simulink model "simulink_audiotest"  (Simulink 7.6)
settings: Solver=ode3  StartTime=0.0  StopTime=100.0  RelTol=1e-3
libraries: dspsrcs4 x3, dspsnks4 x2, simulink x1
settings Model: Creator=KBE  LastModifiedBy=kbe
settings OptimizationCC: InitFltsAndDblsToZero=on
settings DebuggingCC: StrictBusMsg=Warning

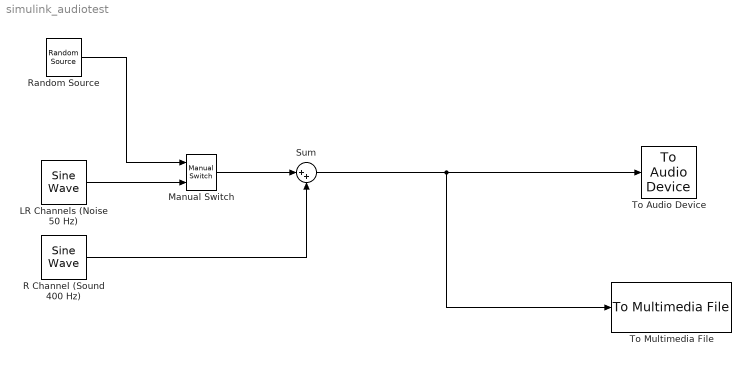
== system simulink_audiotest ==
  LR Channels (Noise 50 Hz) : dspsrcs4/Sine Wave  Amplitude=[1 1]  Frequency=[100 100]  Phase=[0 0]  SampleMode=Discrete  OutComplex=Real  CompMethod=Trigonometric fcn  TableSize=Speed  SampleTime=1/1000  SamplesPerFrame=1  ResetState=Restart at time zero  dataType=double  wordLen=16  udDataType=sfix(16)  fracBitsMode=Best precision  numFracBits=15  OutDataTypeStr=double  LastOutDataTypeStr=double
  Manual Switch : simulink/Signal Routing/Manual Switch  SystemSampleTime=-1  sw=0  action=0  varsize=off
  R Channel (Sound 400 Hz) : dspsrcs4/Sine Wave  Amplitude=[0 1]  Frequency=[400 400]  Phase=[0 0]  SampleMode=Discrete  OutComplex=Real  CompMethod=Trigonometric fcn  TableSize=Speed  SampleTime=1/1000  SamplesPerFrame=1  ResetState=Restart at time zero  dataType=double  wordLen=16  udDataType=sfix(16)  fracBitsMode=Best precision  numFracBits=15  OutDataTypeStr=double  LastOutDataTypeStr=double
  Random Source : dspsrcs4/Random Source  SrcType=Gaussian  NormMethod=Ziggurat  CltLength=12  MinVal=0  MaxVal=1  MeanVal=0  VarVal=1  RepMode=Not repeatable  rawSeed=1  IsInherit=off  SampMode=Discrete  SampTime=1/1000  SampFrame=1  DataType=Double  OutComplex=Real
  Sum : Sum  Inputs=|++
  To Audio Device : dspsnks4/To Audio Device  DialogController=dspDDGCreate  DialogControllerArgs=DataTag1  deviceName=Default  inheritSampleRate=on  sampleRate=44100  deviceDatatype=Determine from input data type  autoBufferSize=on  bufferSize=4096  queueDuration=1.0
  To Multimedia File : dspsnks4/To Multimedia File  DialogController=dspDDGCreate  DialogControllerArgs=DataTag2  outputFilename=TestSound.avi  streamSelection=Audio only  videoCompressor=None (uncompressed)  audioCompressor=None (uncompressed)  imagePorts=Separate color signals  fileType=AVI  audioDatatype=Determine from input data type  fourcc=RGB
  wires:
  Sum/1 -> To Audio Device/1, To Multimedia File/1
  R Channel (Sound 400 Hz)/1 -> Sum/2
  Manual Switch/1 -> Sum/1
  Random Source/1 -> Manual Switch/1
  LR Channels (Noise 50 Hz)/1 -> Manual Switch/2
